simulink model "controlledsystem"  (R2018b)
settings: Solver=ode45  StartTime=0.0  StopTime=30  RelTol=1e-3
libraries: simulink x2
settings Model: Creator=ASUS  LastModifiedBy=ASUS
settings DataIOCC: LimitDataPoints=on  SaveFormat=Array
settings OptimizationCC: BlockReduction=off  BooleanDataType=off  LifeSpan=inf
settings DebuggingCC: SaveWithParameterizedLinksMsg=none  UnderspecifiedInitializationDetection=Classic  MergeDetectMultiDrivingBlocksExec=none  SignalResolutionControl=TryResolveAllWithWarning  SFUnexpectedBacktrackingDiag=warning  SFNoUnconditionalDefaultTransitionDiag=warning  SFExecutionAtInitializationDiag=none
settings HardwareCC: ProdBitPerPointer=32  ProdBitPerSizeT=32  ProdBitPerPtrDiffT=32  ProdLargestAtomicFloat=None  ProdIntDivRoundTo=Undefined  ProdEndianess=Unspecified  ProdWordSize=32  ProdHWDeviceType=32-bit Generic  TargetUnknown=on
settings ModelReferenceCC: PropagateSignalLabelsOutOfModel=off
settings SFSimCC: SimUseLocalCustomCode=off
settings RTWCC: RTWUseLocalCustomCode=off
settings CodeAppCC: StateflowObjectComments=on
settings GRTTargetCC: TargetLangStandard=C89/C90 (ANSI)  GeneratePreprocessorConditionals=Disable all
settings ConfigComp: CovMetricSettings=dw  CovHtmlReporting=on  CovSaveCumulativeToWorkspaceVar=on  CovSaveSingleToWorkspaceVar=on  CovExternalEMLEnable=off  CovSFcnEnable=off

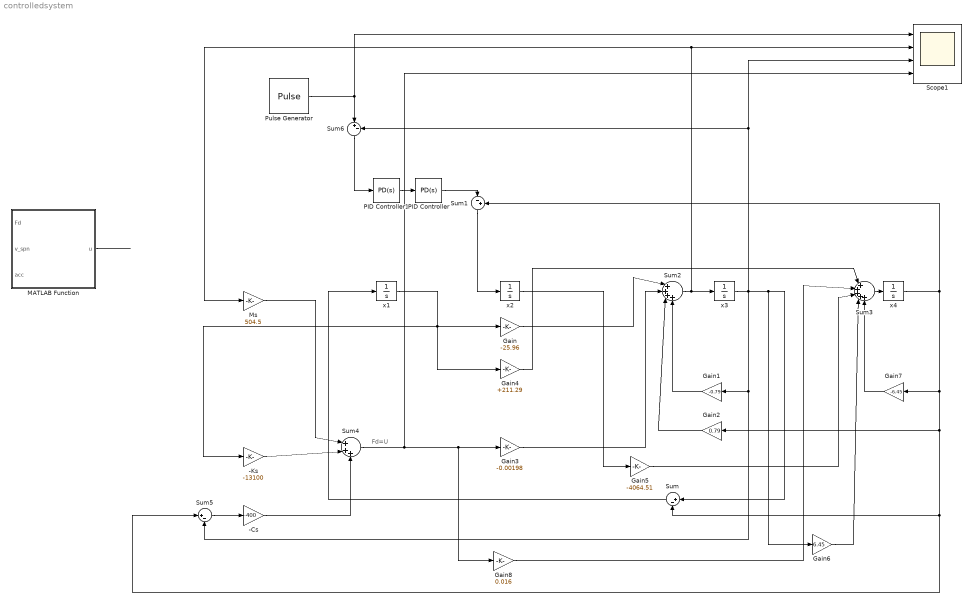
== system controlledsystem ==
  note: Fd=U
  "-Cs " : Gain  Gain=-400
  -Ks : Gain  Gain=-13100
  Gain : Gain  Gain=-25.96
  Gain1 : Gain  Gain=-0.79
  Gain2 : Gain  Gain=0.79
  Gain3 : Gain  Gain=-0.00198
  Gain4 : Gain  Gain=+211.29
  Gain5 : Gain  Gain=-4064.51
  Gain6 : Gain  Gain=6.45
  Gain7 : Gain  Gain=-6.45
  Gain8 : Gain  Gain=0.016
  MATLAB Function : MATLAB Function  TreatAsAtomicUnit=on
  Ms : Gain  Gain=504.5
  PID Controller : simulink/Continuous/PID Controller  Controller=PD  Form=Parallel  TimeDomain=Continuous-time  SampleTime=-1  IntegratorMethod=Forward Euler  FilterMethod=Forward Euler  ControllerParametersSource=internal  P=5.5e-4  I=0  D=5e-4  UseFilter=on  N=100  TunerSelectOption=Transfer Function Based (PID Tuner App)  InitialConditionSource=internal  InitialConditionForIntegrator=0  InitialConditionForFilter=0  DifferentiatorICPrevScaledInput=0  ExternalReset=none  TrackingMode=off  Kt=1  LimitOutput=off  UpperSaturationLimit=inf  LowerSaturationLimit=-inf  LinearizeAsGain=on  AntiWindupMode=none  Kb=1  POutMin=[]  POutMax=[]  IOutMin=[]  IOutMax=[]  DOutMin=[]  DOutMax=[]  NOutMin=[]  NOutMax=[]  SumOutMin=[]  SumOutMax=[]  SaturationOutMin=[]  SaturationOutMax=[]  PParamMin=[]  PParamMax=[]  IParamMin=[]  IParamMax=[]  DParamMin=[]  DParamMax=[]  NParamMin=[]  NParamMax=[]  KbParamMin=[]  KbParamMax=[]  KtParamMin=[]  KtParamMax=[]  KbOutMin=[]  KbOutMax=[]  KtOutMin=[]  KtOutMax=[]  IntegratorOutMin=[]  IntegratorOutMax=[]  FilterOutMin=[]  FilterOutMax=[]  SumI1OutMin=[]  SumI1OutMax=[]  SumI2OutMin=[]  SumI2OutMax=[]  SumI3OutMin=[]  SumI3OutMax=[]  SumI4OutMin=[]  SumI4OutMax=[]  SumDOutMin=[]  SumDOutMax=[]  DifferentiatorOutMin=[]  DifferentiatorOutMax=[]  FilterDiffOutCoefMin=[]  FilterDiffOutCoefMax=[]  ReciprocalOutMin=[]  ReciprocalOutMax=[]  SumDenOutMin=[]  SumDenOutMax=[]  SumNumOutMin=[]  SumNumOutMax=[]  DivideOutMin=[]  DivideOutMax=[]  IntegratorContinuousStateAttributes=''  IntegratorStateMustResolveToSignalObject=off  IntegratorRTWStateStorageClass=Auto  FilterContinuousStateAttributes=''  FilterStateMustResolveToSignalObject=off  FilterRTWStateStorageClass=Auto  ParallelPVariant=InternalParameters  IdealPVariant=Disabled  IVariant=Disabled  DVariant=InternalParameters  IntegratorVariant=Disabled  SatVariant=Disabled  AWVariant=Disabled  PCopyVariant=Disabled  TRVariant=Disabled  FdbkBlocksVariant=Forward  IdealPFdbkVariant=Disabled  SatFdbkVariant=Disabled  DerivativeFilterVariant=ContFilter  NVariant=InternalParameters  NCopyVariant=Disabled  FilterICVariant=InternalICsFilter  IntegratorICVariant=Disabled  ExternalResetVariant=Disabled  TRSumVariant=Passthrough  SumFdbkVariant=Disabled  SumVariant=Sum_PD
  PID Controller1 : simulink/Continuous/PID Controller  Controller=PD  Form=Parallel  TimeDomain=Continuous-time  SampleTime=-1  IntegratorMethod=Forward Euler  FilterMethod=Forward Euler  ControllerParametersSource=internal  P=1.1  I=0  D=1  UseFilter=on  N=100  TunerSelectOption=Transfer Function Based (PID Tuner App)  InitialConditionSource=internal  InitialConditionForIntegrator=0  InitialConditionForFilter=0  DifferentiatorICPrevScaledInput=0  ExternalReset=none  TrackingMode=off  Kt=1  LimitOutput=off  UpperSaturationLimit=inf  LowerSaturationLimit=-inf  LinearizeAsGain=on  AntiWindupMode=none  Kb=1  POutMin=[]  POutMax=[]  IOutMin=[]  IOutMax=[]  DOutMin=[]  DOutMax=[]  NOutMin=[]  NOutMax=[]  SumOutMin=[]  SumOutMax=[]  SaturationOutMin=[]  SaturationOutMax=[]  PParamMin=[]  PParamMax=[]  IParamMin=[]  IParamMax=[]  DParamMin=[]  DParamMax=[]  NParamMin=[]  NParamMax=[]  KbParamMin=[]  KbParamMax=[]  KtParamMin=[]  KtParamMax=[]  KbOutMin=[]  KbOutMax=[]  KtOutMin=[]  KtOutMax=[]  IntegratorOutMin=[]  IntegratorOutMax=[]  FilterOutMin=[]  FilterOutMax=[]  SumI1OutMin=[]  SumI1OutMax=[]  SumI2OutMin=[]  SumI2OutMax=[]  SumI3OutMin=[]  SumI3OutMax=[]  SumI4OutMin=[]  SumI4OutMax=[]  SumDOutMin=[]  SumDOutMax=[]  DifferentiatorOutMin=[]  DifferentiatorOutMax=[]  FilterDiffOutCoefMin=[]  FilterDiffOutCoefMax=[]  ReciprocalOutMin=[]  ReciprocalOutMax=[]  SumDenOutMin=[]  SumDenOutMax=[]  SumNumOutMin=[]  SumNumOutMax=[]  DivideOutMin=[]  DivideOutMax=[]  IntegratorContinuousStateAttributes=''  IntegratorStateMustResolveToSignalObject=off  IntegratorRTWStateStorageClass=Auto  FilterContinuousStateAttributes=''  FilterStateMustResolveToSignalObject=off  FilterRTWStateStorageClass=Auto  ParallelPVariant=InternalParameters  IdealPVariant=Disabled  IVariant=Disabled  DVariant=InternalParameters  IntegratorVariant=Disabled  SatVariant=Disabled  AWVariant=Disabled  PCopyVariant=Disabled  TRVariant=Disabled  FdbkBlocksVariant=Forward  IdealPFdbkVariant=Disabled  SatFdbkVariant=Disabled  DerivativeFilterVariant=ContFilter  NVariant=InternalParameters  NCopyVariant=Disabled  FilterICVariant=InternalICsFilter  IntegratorICVariant=Disabled  ExternalResetVariant=Disabled  TRSumVariant=Passthrough  SumFdbkVariant=Disabled  SumVariant=Sum_PD
  Pulse Generator : DiscretePulseGenerator  PulseType=Time based  Period=15  PulseWidth=15
  Scope1 : Scope  NumInputPorts=4
  Sum : Sum  Inputs=|+-
  Sum1 : Sum  Inputs=|-+
  Sum2 : Sum  Inputs=|++++
  Sum3 : Sum  Inputs=|+++++
  Sum4 : Sum  Inputs=|+++
  Sum5 : Sum  Inputs=|+-
  Sum6 : Sum  Inputs=|+-
  x{1..4} (4 alike) : Integrator
  wires:
  Sum/1 -> x1/1
  x1/1 -> Gain4/1, Gain/1, -Ks/1
  x2/1 -> Gain5/1
  Sum3/1 -> x4/1
  x4/1 -> Sum5/1, Sum/2, Gain2/1, Gain7/1, Sum1/2
  Gain/1 -> Sum2/1
  Gain3/1 -> Sum2/2
  Gain2/1 -> Sum2/3
  Gain1/1 -> Sum2/4
  Gain4/1 -> Sum3/1
  Gain8/1 -> Sum3/2
  Gain5/1 -> Sum3/3
  Gain6/1 -> Sum3/4
  Gain7/1 -> Sum3/5
  Sum4/1 -> Scope1/4, Gain8/1, Gain3/1
  x3/1 -> Gain1/1, Sum5/2, Sum6/2, Scope1/3, Gain6/1, Sum/1
  Sum1/1 -> x2/1
  Sum2/1 -> Ms/1, Scope1/2, x3/1
  Sum5/1 -> "-Cs "/1
  Ms/1 -> Sum4/1
  -Ks/1 -> Sum4/2
  "-Cs "/1 -> Sum4/3
  Pulse Generator/1 -> Sum6/1, Scope1/1
  PID Controller/1 -> Sum1/1
  PID Controller1/1 -> PID Controller/1
  Sum6/1 -> PID Controller1/1
  ? -> MATLAB Function/1(Fd)
  ? -> MATLAB Function/2(v_spn)
  ? -> MATLAB Function/3(acc)
  MATLAB Function/1(u) -> ?

== matlab function controlledsystem/MATLAB Function ==
  data: Fd input; u output; v_spn input; acc input
function u = fcn(Fd,v_spn,acc)

if acc>0
    b=[-165.66 114.63 0.85 -7.39 -0.02 0.29 -8.16e-6 -5.9e-3 5.15e-6 5.65e-5 -3.37e-8 -2.05e-7];
    c=[-535.57 530.84 86.52 -21.73 -4.69 0.64 0.11 -0.01 -1.2e-3 8.34e-5 4.63e-6 -2.69e-7];
    temp1=0;
    temp2=0;
    for i=1:12
        temp1=temp1+b(i).*(v_spn).^(i-1);
        temp2=temp2+c(i).*(v_spn).^(i-1);
    end
    u=(Fd - temp1)/(temp2);
elseif acc<0
    b=[-91.80 121.49 -6.95 -7.06 0.45 0.26 -0.01 -5.1e-3 1.34e-4 4.71e-5 -5.51e-7 -1.68e-7];
    c=[473.89 560.46 -76.17 -26.41 4.01 0.89 -0.09 -0.02 9.98e-4 1.49e-4 -3.96e-6 -5.32e-7];
    temp1=0;
    temp2=0;
    for i=1:12
        temp1=temp1+b(i).*(v_spn).^(i-1);
        temp2=temp2+c(i).*(v_spn).^(i-1);
    end
    u=(Fd - temp1)/(temp2);
else
    u=0;
end
